simulink model "Fixed_Channel_Model_20_Channels"  (R2023a)
settings: Solver=ode23tb  StartTime=0.0  StopTime=3  RelTol=1e-3
libraries: dspfdesign x21, dspsrcs4 x20, dspvision x2
settings Model: Creator=zacha  LastModifiedBy=zacha
settings DebuggingCC: UnconnectedInputMsg=warning  UnconnectedOutputMsg=warning  UnconnectedLineMsg=warning
settings ModelReferenceCC: EnableRefExpFcnMdlSchedulingChecks=on
settings RTWCC: DLArmComputeVersion=19.05

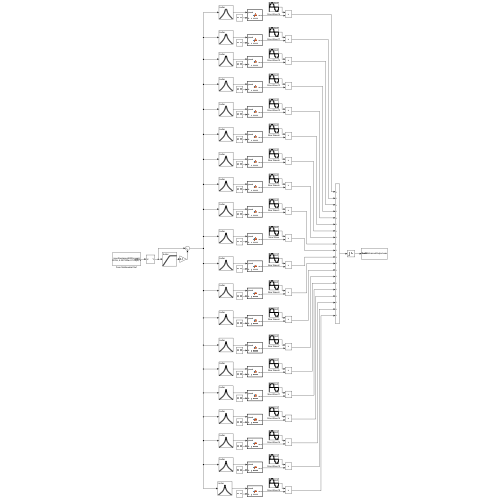
[thumbnail: Simulink's stored preview of the top-level diagram]
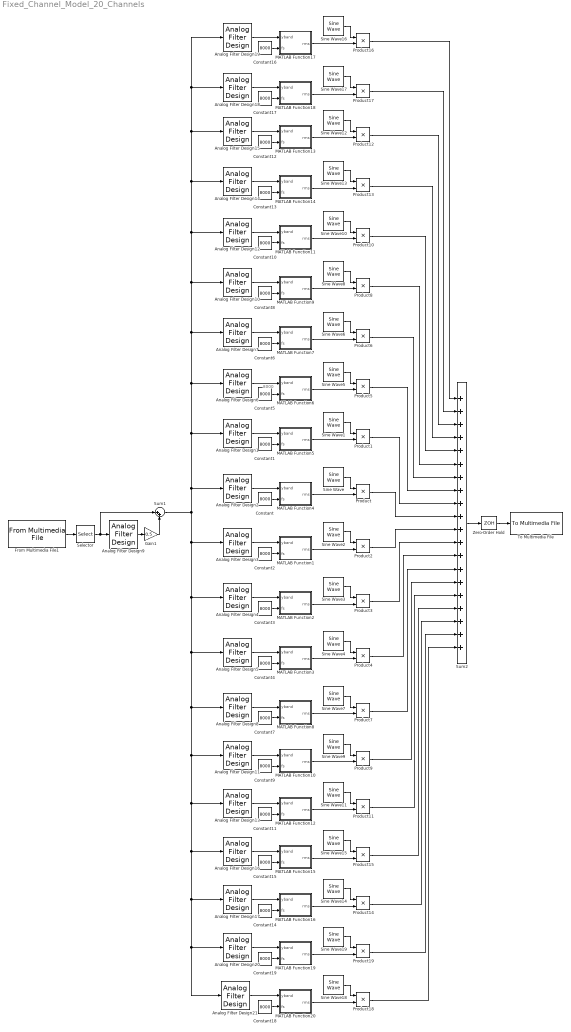
== system Fixed_Channel_Model_20_Channels ==
  note: 8000
  Analog Filter Design1 : dspfdesign/Analog Filter Design  method=Butterworth  filttype=Bandpass  N=6  Wlo=8901.71649069657  Whi=10265.4061283531  Rp=2  Rs=40
  Analog Filter Design10 : dspfdesign/Analog Filter Design  method=Butterworth  filttype=Bandpass  N=6  Wlo=5497.89355477605  Whi=6528.32142910693  Rp=2  Rs=40
  Analog Filter Design11 : dspfdesign/Analog Filter Design  method=Butterworth  filttype=Bandpass  N=6  Wlo=19368.0065720074  Whi=21756.4305609036  Rp=2  Rs=40
  Analog Filter Design12 : dspfdesign/Analog Filter Design  method=Butterworth  filttype=Bandpass  N=6  Wlo=4559.35608112265  Whi=5497.89355477605  Rp=2  Rs=40
  Analog Filter Design13 : dspfdesign/Analog Filter Design  method=Butterworth  filttype=Bandpass  N=6  Wlo=21756.4305609036  Whi=24378.7005532769  Rp=2  Rs=40
  Analog Filter Design14 : dspfdesign/Analog Filter Design  method=Butterworth  filttype=Bandpass  N=6  Wlo=3704.51450375974  Whi=4559.35608112265  Rp=2  Rs=40
  Analog Filter Design15 : dspfdesign/Analog Filter Design  method=Butterworth  filttype=Bandpass  N=6  Wlo=2925.90507909423  Whi=3704.51450375974  Rp=2  Rs=40
  Analog Filter Design16 : dspfdesign/Analog Filter Design  method=Butterworth  filttype=Bandpass  N=6  Wlo=24378.7005532769  Whi=27257.7119620007  Rp=2  Rs=40
  Analog Filter Design17 : dspfdesign/Analog Filter Design  method=Butterworth  filttype=Bandpass  N=6  Wlo=27257.7119620007  Whi=30418.6018458298  Rp=2  Rs=40
  Analog Filter Design18 : dspfdesign/Analog Filter Design  method=Butterworth  filttype=Bandpass  N=6  Wlo=2216.72965731829  Whi=2925.90507909423  Rp=2  Rs=40
  Analog Filter Design19 : dspfdesign/Analog Filter Design  method=Butterworth  filttype=Bandpass  N=6  Wlo=1570.79632679490  Whi=2216.72965731829  Rp=2  Rs=40
  Analog Filter Design2 : dspfdesign/Analog Filter Design  method=Butterworth  filttype=Bandpass  N=6  Wlo=10265.4061283531  Whi=11762.6119981492  Rp=2  Rs=40
  Analog Filter Design20 : dspfdesign/Analog Filter Design  method=Butterworth  filttype=Bandpass  N=6  Wlo=30418.6018458298  Whi=33888.9683846419  Rp=2  Rs=40
  Analog Filter Design21 : dspfdesign/Analog Filter Design  method=Butterworth  filttype=Bandpass  N=6  Wlo=33888.9683846419  Whi=37699.1118430775  Rp=2  Rs=40
  Analog Filter Design3 : dspfdesign/Analog Filter Design  method=Butterworth  filttype=Bandpass  N=6  Wlo=11762.6119981492  Whi=13406.4064178267  Rp=2  Rs=40
  Analog Filter Design4 : dspfdesign/Analog Filter Design  method=Butterworth  filttype=Bandpass  N=6  Wlo=13406.4064178267  Whi=15211.1415906396  Rp=2  Rs=40
  Analog Filter Design5 : dspfdesign/Analog Filter Design  method=Butterworth  filttype=Bandpass  N=6  Wlo=15211.1415906396  Whi=17192.5749164852  Rp=2  Rs=40
  Analog Filter Design6 : dspfdesign/Analog Filter Design  method=Butterworth  filttype=Bandpass  N=6  Wlo=7659.63651668133  Whi=8901.71649069657  Rp=2  Rs=40
  Analog Filter Design7 : dspfdesign/Analog Filter Design  method=Butterworth  filttype=Bandpass  N=6  Wlo=6528.32142910693  Whi=7659.63651668133  Rp=2  Rs=40
  Analog Filter Design8 : dspfdesign/Analog Filter Design  method=Butterworth  filttype=Bandpass  N=6  Wlo=17192.5749164852  Whi=19368.0065720074  Rp=2  Rs=40
  Analog Filter Design9 : dspfdesign/Analog Filter Design  method=Butterworth  filttype=Highpass  N=6  Wlo=7539.82236  Whi=80  Rp=2  Rs=40
  Constant{,1..19} (20 alike) : Constant  Value=8000
  From Multimedia File1 : dspvision/From Multimedia File  inputFilename=C:\Users\zacha\Desktop\Cochlear\Media\inputSentance8000hz.mp3  readRange=[1 Inf]  loop=on  numPlays=1  outputStreams=Audio only  videoDataType=single  audioDataType=double  inheritSampleTime=off  userDefinedSampleTime=1/8000  noAudioOutput=off  isIntensityVideo=off  fourcc=RGB  colorVideoFormat=Separate color signals  outputEOF=off  dataOrg=Column-major  audioFrameSize=1  computeAudioFrameSize=off  outSamplingMode=Sample based
      settings: LibrarySourceBlock=dspsrcs4/From Multimedia File
  Gain1 : Gain  Gain=0.5
  MATLAB Function1 : MATLAB Function  TreatAsAtomicUnit=on
  MATLAB Function10 : MATLAB Function  TreatAsAtomicUnit=on
  MATLAB Function11 : MATLAB Function  TreatAsAtomicUnit=on
  MATLAB Function12 : MATLAB Function  TreatAsAtomicUnit=on
  MATLAB Function13 : MATLAB Function  TreatAsAtomicUnit=on
  MATLAB Function14 : MATLAB Function  TreatAsAtomicUnit=on
  MATLAB Function15 : MATLAB Function  TreatAsAtomicUnit=on
  MATLAB Function16 : MATLAB Function  TreatAsAtomicUnit=on
  MATLAB Function17 : MATLAB Function  TreatAsAtomicUnit=on
  MATLAB Function18 : MATLAB Function  TreatAsAtomicUnit=on
  MATLAB Function19 : MATLAB Function  TreatAsAtomicUnit=on
  MATLAB Function2 : MATLAB Function  TreatAsAtomicUnit=on
  MATLAB Function20 : MATLAB Function  TreatAsAtomicUnit=on
  MATLAB Function3 : MATLAB Function  TreatAsAtomicUnit=on
  MATLAB Function4 : MATLAB Function  TreatAsAtomicUnit=on
  MATLAB Function5 : MATLAB Function  TreatAsAtomicUnit=on
  MATLAB Function6 : MATLAB Function  TreatAsAtomicUnit=on
  MATLAB Function7 : MATLAB Function  TreatAsAtomicUnit=on
  MATLAB Function8 : MATLAB Function  TreatAsAtomicUnit=on
  MATLAB Function9 : MATLAB Function  TreatAsAtomicUnit=on
  Product{,1..19} (20 alike) : Product
  Selector : Selector  NumberOfDimensions=2  InputPortWidth=3  IndexOptions=Select all,Index vector (dialog)  Indices=[2],1  OutputSizes=1,1
  Sine Wave : dspsrcs4/Sine Wave  Amplitude=1  Frequency=1752.93398567535  Phase=0  SampleMode=Discrete  OutComplex=Real  CompMethod=Trigonometric fcn  TableSize=Speed  SampleTime=1/8000  SamplesPerFrame=1  ResetState=Restart at time zero  OutputFrames=off  dataType=double  wordLen=16  udDataType=sfix(16)  fracBitsMode=Best precision  numFracBits=15  OutDataTypeStr=double  LastOutDataTypeStr=double
  Sine Wave1 : dspsrcs4/Sine Wave  Amplitude=1  Frequency=1525.27115483511  Phase=0  SampleMode=Discrete  OutComplex=Real  CompMethod=Trigonometric fcn  TableSize=Speed  SampleTime=1/8000  SamplesPerFrame=1  ResetState=Restart at time zero  OutputFrames=off  dataType=double  wordLen=16  udDataType=sfix(16)  fracBitsMode=Best precision  numFracBits=15  OutDataTypeStr=double  LastOutDataTypeStr=double
  Sine Wave10 : dspsrcs4/Sine Wave  Amplitude=1  Frequency=800.330496731221  Phase=0  SampleMode=Discrete  OutComplex=Real  CompMethod=Trigonometric fcn  TableSize=Speed  SampleTime=1/8000  SamplesPerFrame=1  ResetState=Restart at time zero  OutputFrames=off  dataType=double  wordLen=16  udDataType=sfix(16)  fracBitsMode=Best precision  numFracBits=15  OutDataTypeStr=double  LastOutDataTypeStr=double
  Sine Wave11 : dspsrcs4/Sine Wave  Amplitude=1  Frequency=3671.31708350727  Phase=0  SampleMode=Discrete  OutComplex=Real  CompMethod=Trigonometric fcn  TableSize=Speed  SampleTime=1/8000  SamplesPerFrame=1  ResetState=Restart at time zero  OutputFrames=off  dataType=double  wordLen=16  udDataType=sfix(16)  fracBitsMode=Best precision  numFracBits=15  OutDataTypeStr=double  LastOutDataTypeStr=double
  Sine Wave12 : dspsrcs4/Sine Wave  Amplitude=1  Frequency=527.632025692257  Phase=0  SampleMode=Discrete  OutComplex=Real  CompMethod=Trigonometric fcn  TableSize=Speed  SampleTime=1/8000  SamplesPerFrame=1  ResetState=Restart at time zero  OutputFrames=off  dataType=double  wordLen=16  udDataType=sfix(16)  fracBitsMode=Best precision  numFracBits=15  OutDataTypeStr=double  LastOutDataTypeStr=double
  Sine Wave13 : dspsrcs4/Sine Wave  Amplitude=1  Frequency=657.617926327872  Phase=0  SampleMode=Discrete  OutComplex=Real  CompMethod=Trigonometric fcn  TableSize=Speed  SampleTime=1/8000  SamplesPerFrame=1  ResetState=Restart at time zero  OutputFrames=off  dataType=double  wordLen=16  udDataType=sfix(16)  fracBitsMode=Best precision  numFracBits=15  OutDataTypeStr=double  LastOutDataTypeStr=double
  Sine Wave14 : dspsrcs4/Sine Wave  Amplitude=1  Frequency=4589.73522091778  Phase=0  SampleMode=Discrete  OutComplex=Real  CompMethod=Trigonometric fcn  TableSize=Speed  SampleTime=1/8000  SamplesPerFrame=1  ResetState=Restart at time zero  OutputFrames=off  dataType=double  wordLen=16  udDataType=sfix(16)  fracBitsMode=Best precision  numFracBits=15  OutDataTypeStr=double  LastOutDataTypeStr=double
  Sine Wave15 : dspsrcs4/Sine Wave  Amplitude=1  Frequency=4109.09514766932  Phase=0  SampleMode=Discrete  OutComplex=Real  CompMethod=Trigonometric fcn  TableSize=Speed  SampleTime=1/8000  SamplesPerFrame=1  ResetState=Restart at time zero  OutputFrames=off  dataType=double  wordLen=16  udDataType=sfix(16)  fracBitsMode=Best precision  numFracBits=15  OutDataTypeStr=double  LastOutDataTypeStr=double
  Sine Wave16 : dspsrcs4/Sine Wave  Amplitude=1  Frequency=301.401741230304  Phase=0  SampleMode=Discrete  OutComplex=Real  CompMethod=Trigonometric fcn  TableSize=Speed  SampleTime=1/8000  SamplesPerFrame=1  ResetState=Restart at time zero  OutputFrames=off  dataType=double  wordLen=16  udDataType=sfix(16)  fracBitsMode=Best precision  numFracBits=15  OutDataTypeStr=double  LastOutDataTypeStr=double
  Sine Wave17 : dspsrcs4/Sine Wave  Amplitude=1  Frequency=409.237869408070  Phase=0  SampleMode=Discrete  OutComplex=Real  CompMethod=Trigonometric fcn  TableSize=Speed  SampleTime=1/8000  SamplesPerFrame=1  ResetState=Restart at time zero  OutputFrames=off  dataType=double  wordLen=16  udDataType=sfix(16)  fracBitsMode=Best precision  numFracBits=15  OutDataTypeStr=double  LastOutDataTypeStr=double
  Sine Wave18 : dspsrcs4/Sine Wave  Amplitude=1  Frequency=5696.79841735036  Phase=0  SampleMode=Discrete  OutComplex=Real  CompMethod=Trigonometric fcn  TableSize=Speed  SampleTime=1/8000  SamplesPerFrame=1  ResetState=Restart at time zero  OutputFrames=off  dataType=double  wordLen=16  udDataType=sfix(16)  fracBitsMode=Best precision  numFracBits=15  OutDataTypeStr=double  LastOutDataTypeStr=double
  Sine Wave19 : dspsrcs4/Sine Wave  Amplitude=1  Frequency=5117.43384020440  Phase=0  SampleMode=Discrete  OutComplex=Real  CompMethod=Trigonometric fcn  TableSize=Speed  SampleTime=1/8000  SamplesPerFrame=1  ResetState=Restart at time zero  OutputFrames=off  dataType=double  wordLen=16  udDataType=sfix(16)  fracBitsMode=Best precision  numFracBits=15  OutDataTypeStr=double  LastOutDataTypeStr=double
  Sine Wave2 : dspsrcs4/Sine Wave  Amplitude=1  Frequency=2002.88684683675  Phase=0  SampleMode=Discrete  OutComplex=Real  CompMethod=Trigonometric fcn  TableSize=Speed  SampleTime=1/8000  SamplesPerFrame=1  ResetState=Restart at time zero  OutputFrames=off  dataType=double  wordLen=16  udDataType=sfix(16)  fracBitsMode=Best precision  numFracBits=15  OutDataTypeStr=double  LastOutDataTypeStr=double
  Sine Wave3 : dspsrcs4/Sine Wave  Amplitude=1  Frequency=2277.31211235852  Phase=0  SampleMode=Discrete  OutComplex=Real  CompMethod=Trigonometric fcn  TableSize=Speed  SampleTime=1/8000  SamplesPerFrame=1  ResetState=Restart at time zero  OutputFrames=off  dataType=double  wordLen=16  udDataType=sfix(16)  fracBitsMode=Best precision  numFracBits=15  OutDataTypeStr=double  LastOutDataTypeStr=double
  Sine Wave4 : dspsrcs4/Sine Wave  Amplitude=1  Frequency=2578.60582832868  Phase=0  SampleMode=Discrete  OutComplex=Real  CompMethod=Trigonometric fcn  TableSize=Speed  SampleTime=1/8000  SamplesPerFrame=1  ResetState=Restart at time zero  OutputFrames=off  dataType=double  wordLen=16  udDataType=sfix(16)  fracBitsMode=Best precision  numFracBits=15  OutDataTypeStr=double  LastOutDataTypeStr=double
  Sine Wave5 : dspsrcs4/Sine Wave  Amplitude=1  Frequency=1317.91059770701  Phase=0  SampleMode=Discrete  OutComplex=Real  CompMethod=Trigonometric fcn  TableSize=Speed  SampleTime=1/8000  SamplesPerFrame=1  ResetState=Restart at time zero  OutputFrames=off  dataType=double  wordLen=16  udDataType=sfix(16)  fracBitsMode=Best precision  numFracBits=15  OutDataTypeStr=double  LastOutDataTypeStr=double
  Sine Wave6 : dspsrcs4/Sine Wave  Amplitude=1  Frequency=1129.04181972607  Phase=0  SampleMode=Discrete  OutComplex=Real  CompMethod=Trigonometric fcn  TableSize=Speed  SampleTime=1/8000  SamplesPerFrame=1  ResetState=Restart at time zero  OutputFrames=off  dataType=double  wordLen=16  udDataType=sfix(16)  fracBitsMode=Best precision  numFracBits=15  OutDataTypeStr=double  LastOutDataTypeStr=double
  Sine Wave7 : dspsrcs4/Sine Wave  Amplitude=1  Frequency=2909.39863310382  Phase=0  SampleMode=Discrete  OutComplex=Real  CompMethod=Trigonometric fcn  TableSize=Speed  SampleTime=1/8000  SamplesPerFrame=1  ResetState=Restart at time zero  OutputFrames=off  dataType=double  wordLen=16  udDataType=sfix(16)  fracBitsMode=Best precision  numFracBits=15  OutDataTypeStr=double  LastOutDataTypeStr=double
  Sine Wave8 : dspsrcs4/Sine Wave  Amplitude=1  Frequency=957.015780685397  Phase=0  SampleMode=Discrete  OutComplex=Real  CompMethod=Trigonometric fcn  TableSize=Speed  SampleTime=1/8000  SamplesPerFrame=1  ResetState=Restart at time zero  OutputFrames=off  dataType=double  wordLen=16  udDataType=sfix(16)  fracBitsMode=Best precision  numFracBits=15  OutDataTypeStr=double  LastOutDataTypeStr=double
  Sine Wave9 : dspsrcs4/Sine Wave  Amplitude=1  Frequency=3272.57872578734  Phase=0  SampleMode=Discrete  OutComplex=Real  CompMethod=Trigonometric fcn  TableSize=Speed  SampleTime=1/8000  SamplesPerFrame=1  ResetState=Restart at time zero  OutputFrames=off  dataType=double  wordLen=16  udDataType=sfix(16)  fracBitsMode=Best precision  numFracBits=15  OutDataTypeStr=double  LastOutDataTypeStr=double
  Sum1 : Sum  Inputs=|++
  Sum2 : Sum  Inputs=20
  To Multimedia File : dspvision/To Multimedia File  outputFilename=C:\Users\zacha\Desktop\Cochlear\Media\fixed20channelOutput.wav  streamSelection=Audio only  videoCompressor=None (uncompressed)  audioCompressor=None (uncompressed)  imagePorts=Separate color signals  fileType=WAV  audioDatatype=16-bit integer  fourcc=RGB  videoQuality=75  mj2000CompFactor=10
      settings: LibrarySourceBlock=dspsnks4/To Multimedia File
  Zero-Order Hold : ZeroOrderHold  SampleTime=-1
  wires:
  Analog Filter Design2/1 -> MATLAB Function4/1(yband)
  Constant/1 -> MATLAB Function4/2(fs)
  MATLAB Function4/1(rms) -> Product/2
  Sine Wave/1 -> Product/1
  Sine Wave1/1 -> Product1/1
  Analog Filter Design1/1 -> MATLAB Function5/1(yband)
  MATLAB Function5/1(rms) -> Product1/2
  Constant1/1 -> MATLAB Function5/2(fs)
  Sine Wave2/1 -> Product2/1
  Analog Filter Design3/1 -> MATLAB Function1/1(yband)
  MATLAB Function1/1(rms) -> Product2/2
  Constant2/1 -> MATLAB Function1/2(fs)
  Sine Wave3/1 -> Product3/1
  MATLAB Function2/1(rms) -> Product3/2
  Analog Filter Design4/1 -> MATLAB Function2/1(yband)
  Constant3/1 -> MATLAB Function2/2(fs)
  Sine Wave4/1 -> Product4/1
  MATLAB Function3/1(rms) -> Product4/2
  Analog Filter Design5/1 -> MATLAB Function3/1(yband)
  Constant4/1 -> MATLAB Function3/2(fs)
  Sine Wave5/1 -> Product5/1
  MATLAB Function6/1(rms) -> Product5/2
  Analog Filter Design6/1 -> MATLAB Function6/1(yband)
  Constant5/1 -> MATLAB Function6/2(fs)
  Product/1 -> Sum2/10
  Product2/1 -> Sum2/11
  Product1/1 -> Sum2/9
  Product5/1 -> Sum2/8
  Product3/1 -> Sum2/12
  Product4/1 -> Sum2/13
  Constant6/1 -> MATLAB Function7/2(fs)
  MATLAB Function7/1(rms) -> Product6/2
  Analog Filter Design7/1 -> MATLAB Function7/1(yband)
  Sine Wave6/1 -> Product6/1
  Product6/1 -> Sum2/7
  Constant7/1 -> MATLAB Function8/2(fs)
  MATLAB Function8/1(rms) -> Product7/2
  Analog Filter Design8/1 -> MATLAB Function8/1(yband)
  Sine Wave7/1 -> Product7/1
  Product7/1 -> Sum2/14
  Gain1/1 -> Sum1/2
  Selector/1 -> Analog Filter Design9/1, Sum1/1
  From Multimedia File1/1 -> Selector/1
  Analog Filter Design9/1 -> Gain1/1
  MATLAB Function9/1(rms) -> Product8/2
  Analog Filter Design10/1 -> MATLAB Function9/1(yband)
  Product8/1 -> Sum2/6
  Sine Wave8/1 -> Product8/1
  Constant8/1 -> MATLAB Function9/2(fs)
  MATLAB Function10/1(rms) -> Product9/2
  Analog Filter Design11/1 -> MATLAB Function10/1(yband)
  Sine Wave9/1 -> Product9/1
  Constant9/1 -> MATLAB Function10/2(fs)
  Product9/1 -> Sum2/15
  Constant10/1 -> MATLAB Function11/2(fs)
  Sine Wave10/1 -> Product10/1
  Analog Filter Design12/1 -> MATLAB Function11/1(yband)
  MATLAB Function11/1(rms) -> Product10/2
  Sine Wave11/1 -> Product11/1
  Analog Filter Design13/1 -> MATLAB Function12/1(yband)
  MATLAB Function12/1(rms) -> Product11/2
  Constant11/1 -> MATLAB Function12/2(fs)
  Product11/1 -> Sum2/16
  Product10/1 -> Sum2/5
  MATLAB Function13/1(rms) -> Product12/2
  Analog Filter Design15/1 -> MATLAB Function13/1(yband)
  Sine Wave12/1 -> Product12/1
  Constant12/1 -> MATLAB Function13/2(fs)
  Constant13/1 -> MATLAB Function14/2(fs)
  Sine Wave13/1 -> Product13/1
  Analog Filter Design14/1 -> MATLAB Function14/1(yband)
  MATLAB Function14/1(rms) -> Product13/2
  Sine Wave15/1 -> Product15/1
  Analog Filter Design16/1 -> MATLAB Function15/1(yband)
  Sine Wave14/1 -> Product14/1
  Constant14/1 -> MATLAB Function16/2(fs)
  Analog Filter Design17/1 -> MATLAB Function16/1(yband)
  MATLAB Function15/1(rms) -> Product15/2
  Constant15/1 -> MATLAB Function15/2(fs)
  MATLAB Function16/1(rms) -> Product14/2
  Product15/1 -> Sum2/17
  Product14/1 -> Sum2/18
  Product13/1 -> Sum2/4
  Product12/1 -> Sum2/3
  Sum2/1 -> Zero-Order Hold/1
  Zero-Order Hold/1 -> To Multimedia File/1
  MATLAB Function18/1(rms) -> Product17/2
  Constant17/1 -> MATLAB Function18/2(fs)
  Analog Filter Design18/1 -> MATLAB Function18/1(yband)
  Constant16/1 -> MATLAB Function17/2(fs)
  Sine Wave16/1 -> Product16/1
  MATLAB Function17/1(rms) -> Product16/2
  Sine Wave17/1 -> Product17/1
  Analog Filter Design19/1 -> MATLAB Function17/1(yband)
  Product17/1 -> Sum2/2
  Product16/1 -> Sum2/1
  Analog Filter Design21/1 -> MATLAB Function20/1(yband)
  MATLAB Function19/1(rms) -> Product19/2
  Constant19/1 -> MATLAB Function19/2(fs)
  MATLAB Function20/1(rms) -> Product18/2
  Sine Wave19/1 -> Product19/1
  Constant18/1 -> MATLAB Function20/2(fs)
  Sine Wave18/1 -> Product18/1
  Sum1/1 -> Analog Filter Design19/1, Analog Filter Design18/1, Analog Filter Design15/1, Analog Filter Design14/1, Analog Filter Design12/1, Analog Filter Design10/1, Analog Filter Design7/1, Analog Filter Design6/1, Analog Filter Design1/1, Analog Filter Design2/1, Analog Filter Design21/1, Analog Filter Design20/1, Analog Filter Design17/1, Analog Filter Design16/1, Analog Filter Design13/1, Analog Filter Design11/1, Analog Filter Design8/1, Analog Filter Design5/1, Analog Filter Design4/1, Analog Filter Design3/1
  Analog Filter Design20/1 -> MATLAB Function19/1(yband)
  Product19/1 -> Sum2/19
  Product18/1 -> Sum2/20

== matlab function Fixed_Channel_Model_20_Channels/MATLAB Function13 ==
  data: yband input; rms output; fs input
function rms = getrms(yband,fs)

    y = abs(yband); %rectifying it makes it sound bad

    [b,a] = butter(2,400/(fs/2));

    z = filter(b,a,y); %this filter also makes it sound bad

    windowsize = round(4/(1000/fs)); %rms computed every 4ms = windowsize samples

    [yupper,ylower] = envelope(yband,windowsize,'rms'); %changed to yband here

    %envelope(z,windowsize,'rms');

    rms = yupper;
end

== matlab function Fixed_Channel_Model_20_Channels/MATLAB Function14 ==
  data: yband input; rms output; fs input
function rms = getrms(yband,fs)

    y = abs(yband); %rectifying it makes it sound bad

    [b,a] = butter(2,400/(fs/2));

    z = filter(b,a,y); %this filter also makes it sound bad

    windowsize = round(4/(1000/fs)); %rms computed every 4ms = windowsize samples

    [yupper,ylower] = envelope(yband,windowsize,'rms'); %changed to yband here

    %envelope(z,windowsize,'rms');

    rms = yupper;
end

== matlab function Fixed_Channel_Model_20_Channels/MATLAB Function15 ==
  data: yband input; rms output; fs input
function rms = getrms(yband,fs)

    y = abs(yband); %rectifying it makes it sound bad

    [b,a] = butter(2,400/(fs/2));

    z = filter(b,a,y); %this filter also makes it sound bad

    windowsize = round(4/(1000/fs)); %rms computed every 4ms = windowsize samples

    [yupper,ylower] = envelope(yband,windowsize,'rms'); %changed to yband here

    %envelope(z,windowsize,'rms');

    rms = yupper;
end

== matlab function Fixed_Channel_Model_20_Channels/MATLAB Function16 ==
  data: yband input; rms output; fs input
function rms = getrms(yband,fs)

    y = abs(yband); %rectifying it makes it sound bad

    [b,a] = butter(2,400/(fs/2));

    z = filter(b,a,y); %this filter also makes it sound bad

    windowsize = round(4/(1000/fs)); %rms computed every 4ms = windowsize samples

    [yupper,ylower] = envelope(yband,windowsize,'rms'); %changed to yband here

    %envelope(z,windowsize,'rms');

    rms = yupper;
end

== matlab function Fixed_Channel_Model_20_Channels/MATLAB Function17 ==
  data: yband input; rms output; fs input
function rms = getrms(yband,fs)

    y = abs(yband); %rectifying it makes it sound bad

    [b,a] = butter(2,400/(fs/2));

    z = filter(b,a,y); %this filter also makes it sound bad

    windowsize = round(4/(1000/fs)); %rms computed every 4ms = windowsize samples

    [yupper,ylower] = envelope(yband,windowsize,'rms'); %changed to yband here

    %envelope(z,windowsize,'rms');

    rms = yupper;
end

== matlab function Fixed_Channel_Model_20_Channels/MATLAB Function18 ==
  data: yband input; rms output; fs input
function rms = getrms(yband,fs)

    y = abs(yband); %rectifying it makes it sound bad

    [b,a] = butter(2,400/(fs/2));

    z = filter(b,a,y); %this filter also makes it sound bad

    windowsize = round(4/(1000/fs)); %rms computed every 4ms = windowsize samples

    [yupper,ylower] = envelope(yband,windowsize,'rms'); %changed to yband here

    %envelope(z,windowsize,'rms');

    rms = yupper;
end

== matlab function Fixed_Channel_Model_20_Channels/MATLAB Function19 ==
  data: yband input; rms output; fs input
function rms = getrms(yband,fs)

    y = abs(yband); %rectifying it makes it sound bad

    [b,a] = butter(2,400/(fs/2));

    z = filter(b,a,y); %this filter also makes it sound bad

    windowsize = round(4/(1000/fs)); %rms computed every 4ms = windowsize samples

    [yupper,ylower] = envelope(yband,windowsize,'rms'); %changed to yband here

    %envelope(z,windowsize,'rms');

    rms = yupper;
end

== matlab function Fixed_Channel_Model_20_Channels/MATLAB Function20 ==
  data: yband input; rms output; fs input
function rms = getrms(yband,fs)

    y = abs(yband); %rectifying it makes it sound bad

    [b,a] = butter(2,400/(fs/2));

    z = filter(b,a,y); %this filter also makes it sound bad

    windowsize = round(4/(1000/fs)); %rms computed every 4ms = windowsize samples

    [yupper,ylower] = envelope(yband,windowsize,'rms'); %changed to yband here

    %envelope(z,windowsize,'rms');

    rms = yupper;
end

== matlab function Fixed_Channel_Model_20_Channels/MATLAB Function2 ==
  data: yband input; rms output; fs input
function rms = getrms(yband,fs)

    y = abs(yband); %rectifying it makes it sound bad

    [b,a] = butter(2,400/(fs/2));

    z = filter(b,a,y); %this filter also makes it sound bad

    windowsize = round(4/(1000/fs)); %rms computed every 4ms = windowsize samples

    [yupper,ylower] = envelope(yband,windowsize,'rms'); %changed to yband here

    %envelope(z,windowsize,'rms');

    rms = yupper;
end

== matlab function Fixed_Channel_Model_20_Channels/MATLAB Function3 ==
  data: yband input; rms output; fs input
function rms = getrms(yband,fs)

    y = abs(yband); %rectifying it makes it sound bad

    [b,a] = butter(2,400/(fs/2));

    z = filter(b,a,y); %this filter also makes it sound bad

    windowsize = round(4/(1000/fs)); %rms computed every 4ms = windowsize samples

    [yupper,ylower] = envelope(yband,windowsize,'rms'); %changed to yband here

    %envelope(z,windowsize,'rms');

    rms = yupper;
end

== matlab function Fixed_Channel_Model_20_Channels/MATLAB Function6 ==
  data: yband input; rms output; fs input
function rms = getrms(yband,fs)

    y = abs(yband); %rectifying it makes it sound bad

    [b,a] = butter(2,400/(fs/2));

    z = filter(b,a,y); %this filter also makes it sound bad

    windowsize = round(4/(1000/fs)); %rms computed every 4ms = windowsize samples

    [yupper,ylower] = envelope(yband,windowsize,'rms'); %changed to yband here

    %envelope(z,windowsize,'rms');

    rms = yupper;
end

== matlab function Fixed_Channel_Model_20_Channels/MATLAB Function4 ==
  data: yband input; rms output; fs input
function rms = getrms(yband,fs)

    y = abs(yband); %rectifying it makes it sound bad

    [b,a] = butter(2,400/(fs/2));

    z = filter(b,a,y); %this filter also makes it sound bad

    windowsize = round(4/(1000/fs)); %rms computed every 4ms = windowsize samples

    [yupper,ylower] = envelope(yband,windowsize,'rms'); %changed to yband here

    %envelope(z,windowsize,'rms');

    rms = yupper;
end

== matlab function Fixed_Channel_Model_20_Channels/MATLAB Function5 ==
  data: yband input; rms output; fs input
function rms = getrms(yband,fs)

    y = abs(yband); %rectifying it makes it sound bad

    [b,a] = butter(2,400/(fs/2));

    z = filter(b,a,y); %this filter also makes it sound bad

    windowsize = round(4/(1000/fs)); %rms computed every 4ms = windowsize samples

    [yupper,ylower] = envelope(yband,windowsize,'rms'); %changed to yband here

    %envelope(z,windowsize,'rms');

    rms = yupper;
end

== matlab function Fixed_Channel_Model_20_Channels/MATLAB Function7 ==
  data: yband input; rms output; fs input
function rms = getrms(yband,fs)

    y = abs(yband); %rectifying it makes it sound bad

    [b,a] = butter(2,400/(fs/2));

    z = filter(b,a,y); %this filter also makes it sound bad

    windowsize = round(4/(1000/fs)); %rms computed every 4ms = windowsize samples

    [yupper,ylower] = envelope(yband,windowsize,'rms'); %changed to yband here

    %envelope(z,windowsize,'rms');

    rms = yupper;
end

== matlab function Fixed_Channel_Model_20_Channels/MATLAB Function8 ==
  data: yband input; rms output; fs input
function rms = getrms(yband,fs)

    y = abs(yband); %rectifying it makes it sound bad

    [b,a] = butter(2,400/(fs/2));

    z = filter(b,a,y); %this filter also makes it sound bad

    windowsize = round(4/(1000/fs)); %rms computed every 4ms = windowsize samples

    [yupper,ylower] = envelope(yband,windowsize,'rms'); %changed to yband here

    %envelope(z,windowsize,'rms');

    rms = yupper;
end

== matlab function Fixed_Channel_Model_20_Channels/MATLAB Function9 ==
  data: yband input; rms output; fs input
function rms = getrms(yband,fs)

    y = abs(yband); %rectifying it makes it sound bad

    [b,a] = butter(2,400/(fs/2));

    z = filter(b,a,y); %this filter also makes it sound bad

    windowsize = round(4/(1000/fs)); %rms computed every 4ms = windowsize samples

    [yupper,ylower] = envelope(yband,windowsize,'rms'); %changed to yband here

    %envelope(z,windowsize,'rms');

    rms = yupper;
end

== matlab function Fixed_Channel_Model_20_Channels/MATLAB Function10 ==
  data: yband input; rms output; fs input
function rms = getrms(yband,fs)

    y = abs(yband); %rectifying it makes it sound bad

    [b,a] = butter(2,400/(fs/2));

    z = filter(b,a,y); %this filter also makes it sound bad

    windowsize = round(4/(1000/fs)); %rms computed every 4ms = windowsize samples

    [yupper,ylower] = envelope(yband,windowsize,'rms'); %changed to yband here

    %envelope(z,windowsize,'rms');

    rms = yupper;
end

== matlab function Fixed_Channel_Model_20_Channels/MATLAB Function11 ==
  data: yband input; rms output; fs input
function rms = getrms(yband,fs)

    y = abs(yband); %rectifying it makes it sound bad

    [b,a] = butter(2,400/(fs/2));

    z = filter(b,a,y); %this filter also makes it sound bad

    windowsize = round(4/(1000/fs)); %rms computed every 4ms = windowsize samples

    [yupper,ylower] = envelope(yband,windowsize,'rms'); %changed to yband here

    %envelope(z,windowsize,'rms');

    rms = yupper;
end

== matlab function Fixed_Channel_Model_20_Channels/MATLAB Function1 ==
  data: yband input; rms output; fs input
function rms = getrms(yband,fs)

    y = abs(yband); %rectifying it makes it sound bad

    [b,a] = butter(2,400/(fs/2));

    z = filter(b,a,y); %this filter also makes it sound bad

    windowsize = round(4/(1000/fs)); %rms computed every 4ms = windowsize samples

    [yupper,ylower] = envelope(yband,windowsize,'rms'); %changed to yband here

    %envelope(z,windowsize,'rms');

    rms = yupper;
end

== matlab function Fixed_Channel_Model_20_Channels/MATLAB Function12 ==
  data: yband input; rms output; fs input
function rms = getrms(yband,fs)

    y = abs(yband); %rectifying it makes it sound bad

    [b,a] = butter(2,400/(fs/2));

    z = filter(b,a,y); %this filter also makes it sound bad

    windowsize = round(4/(1000/fs)); %rms computed every 4ms = windowsize samples

    [yupper,ylower] = envelope(yband,windowsize,'rms'); %changed to yband here

    %envelope(z,windowsize,'rms');

    rms = yupper;
end
